simulink model "closedloop"  (R2022a)
settings: Solver=ode4  StartTime=0.0  StopTime=0.07  FixedStep=1e-8  RelTol=1e-3
values from neighbouring files (symbols this model uses):
  d = [1/w_p 1 0]    [code.m]
  Gmb = 1/24.044    (= 0.0415904175678)    [code.m]
  n = [1 w_z]    [code.m]
libraries: spsSeriesRLCBranchLib x3, spsVoltageMeasurementLib x2, spsCurrentMeasurementLib x1, spsDCVoltageSourceLib x1, spsDiodeLib x1, spsMosfetLib x1, simulink x1, spspowerguiLib x1
settings Model: Creator=eee  LastModifiedBy=eee

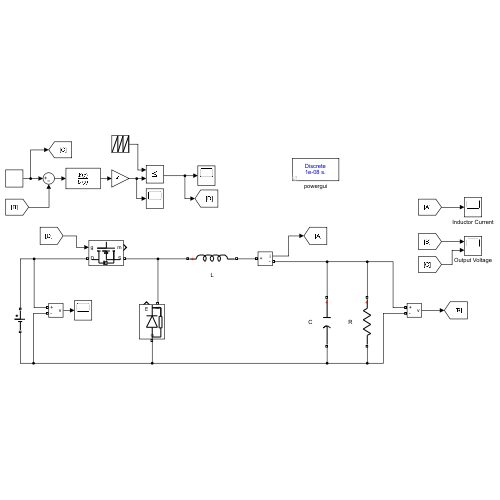
[thumbnail: Simulink's stored preview of the top-level diagram]
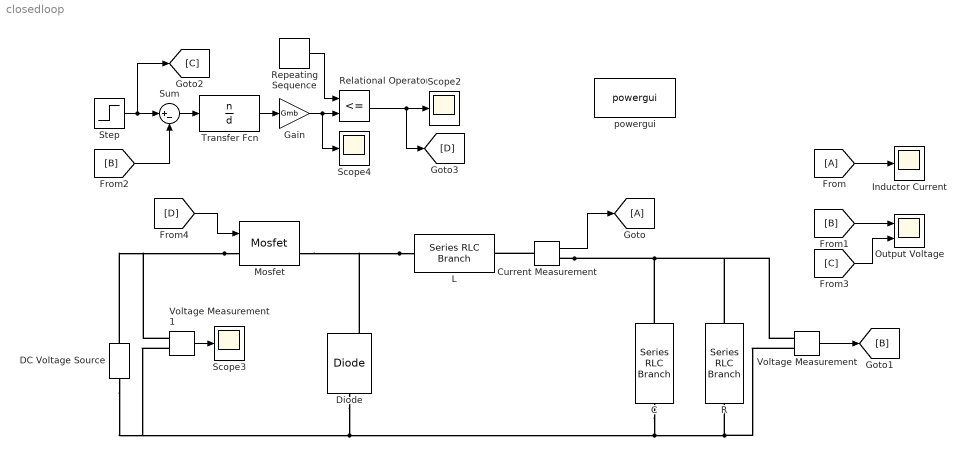
== system closedloop ==
  C : spsSeriesRLCBranchLib/Series RLC Branch  LConnTagsString=__new0  RConnTagsString=__new0  BranchType=C  Resistance=1  Inductance=1e-3  SetiL0=off  InitialCurrent=0  Capacitance=100e-6  Setx0=off  InitialVoltage=0  Measurements=None
  Current Measurement : spsCurrentMeasurementLib/Current Measurement  PhasorSimulation=off  OutputType=Complex  PSBequivalent=0
  DC Voltage Source : spsDCVoltageSourceLib/DC Voltage Source  Amplitude=24  Measurements=None
  Diode : spsDiodeLib/Diode  Ron=0.001  Lon=0  Vf=0.8  IC=0  UseSnubber=0  Rs=500  Cs=250e-9  Measurements=on
  From : From
  Gain : Gain  Gain=Gmb
  Goto : Goto
  Inductor Current : Scope
  L : spsSeriesRLCBranchLib/Series RLC Branch  LConnTagsString=__new0  RConnTagsString=__new0  BranchType=L  Resistance=1  Inductance=50e-6  SetiL0=off  InitialCurrent=0  Capacitance=1e-6  Setx0=off  InitialVoltage=0  Measurements=None
  Mosfet : spsMosfetLib/Mosfet  Ron=0.1  Lon=0  Rd=0.01  Vfd=0  IC=0  Rs=1e5  Cs=inf  Measurements=on
  Output Voltage : Scope  NumInputPorts=2
  R : spsSeriesRLCBranchLib/Series RLC Branch  LConnTagsString=__new0  RConnTagsString=__new0  BranchType=R  Resistance=2  Inductance=1e-3  SetiL0=off  InitialCurrent=0  Capacitance=1e-6  Setx0=off  InitialVoltage=0  Measurements=None
  Relational Operator : RelationalOperator  Operator=<=  OutDataTypeStr=boolean  RndMeth=Simplest  InputSameDT=off
  Repeating Sequence : simulink/Sources/Repeating Sequence  rep_seq_t=[0 1e-5]  rep_seq_y=[0 1]
  Scope2 : Scope
  Scope3 : Scope
  Scope4 : Scope
  Step : Step  Time=0.035  Before=10  After=15
  Sum : Sum  Inputs=|+-
  Transfer Fcn : TransferFcn  Numerator=n  Denominator=d
  Voltage Measurement : spsVoltageMeasurementLib/Voltage Measurement  PhasorSimulation=off  OutputType=Complex  PSBequivalent=0
  Voltage Measurement1 : spsVoltageMeasurementLib/Voltage Measurement  PhasorSimulation=off  OutputType=Complex  PSBequivalent=0
  powergui : spspowerguiLib/powergui  Priority=1  SimulationMode=Discrete  SampleTime=1e-8  frequency=60  Iterations=50  frequencyindice=0  Pbase=100e6  ErrMax=1e-4  UnitsV=kV  UnitsW=MW  buscounter=0  FunctionMessages=off  echomessages=off  EnableUseOfTLC=off  CurrentSourceSwitches=off  DisableSnubberDevices=off  DisableRonSwitches=off  DisableVfSwitches=off  DisplayEquations=off  AutomaticDiscreteSolvers=off  SolverType=Tustin/Backward Euler (TBE)  Interpol=off  ExternalGateDelay=off  methode=off  Ts=100  x0status=blocks  SPID=on  SwTol=0  HookPort=off  NonlinearTolerance=1e-4  nMaxIteration=100  ContinueOnMaxIteration=off  RestoreLinks=warning  ResistiveCurrentMeasurement=off  Frange=[0:2:500]  Ylog=off  Xlog=on  ShowGrid=off  save=off  variable=ZData  structure=0  ZoomFFT=off  StartTime=0.0  cycles=1  DisplayStyle=1  fundamental=60  FreqAxis=off  MaxFrequency=1000  frequencyindicesteady=1  RmsSteady=1  display=off
  wires:
  Current Measurement/1 -> Goto/1
  Repeating Sequence/1 -> Relational Operator/1
  Relational Operator/1 -> [D], Scope2/1
  [B] -> Output Voltage/1
  [C] -> Output Voltage/2
  Voltage Measurement/1 -> [B]
  Voltage Measurement1/1 -> Scope3/1
  From/1 -> Inductor Current/1
  Step/1 -> [C], Sum/1
  Sum/1 -> Transfer Fcn/1
  Transfer Fcn/1 -> Gain/1
  [B] -> Sum/2
  Gain/1 -> Scope4/1, Relational Operator/2
  [D] -> Mosfet/1
  connections:
  Voltage Measurement/LConn2 -- R/RConn1 -- C/RConn1 -- DC Voltage Source/LConn1 -- Voltage Measurement1/LConn2 -- Diode/LConn1
  Current Measurement/RConn1 -- C/LConn1 -- R/LConn1 -- Voltage Measurement/LConn1
  L/LConn1 -- Mosfet/RConn1 -- Diode/RConn1
  Mosfet/LConn1 -- DC Voltage Source/RConn1 -- Voltage Measurement1/LConn1
  Current Measurement/LConn1 -- L/RConn1
